simulink model "Elevator"  (R2023b)
settings: Solver=VariableStepAuto  StartTime=0.0  StopTime=inf  RelTol=1e-3
(part 2 of 2)

== matlab function Elevator/MATLAB Function ==
  data: eb input; i1 input; i2 input; i3 input; EBL output; pw input; o1 input; o2 input; o3 input; EL output; VE output; VD output; i_f input; f_t output; c_f output; f output; i_f output; n_f output; i_2 output; i_3 output; i_1 output
function [EBL,EL,VE,VD,f_t,c_f,f,i_f,n_f,i_2,i_3,i_1] = fcn(eb,i1,i2,i3,pw,o1,o2,o3,i_f)



%-----------------------------------------------------------------------------------
if o1 == 1
    f = 1;
elseif o2 == 1 
    f = 2;
elseif o3 == 1  
    f = 3;
else
    f = 0;
end

%------------------------------------------------------------------------------------
if i1==1 && i2==0 && i3==0
    n_f = 1;
elseif i1==0 && i2==1 && i3==0
    n_f = 2;
elseif i1==0 && i2==0 && i3==1
    n_f = 3;
elseif i1==1 && i2==1 && i3==0
    n_f = 4;
elseif i1==1 && i2==0 && i3==1
    n_f = 5;
elseif i1==0 && i2==1 && i3==1
    n_f = 6;
elseif i1==1 && i2==1 && i3==1
    n_f = 7; 
else
    n_f = 0;
end
%-----------------------------------------------------------------------------------
if eb == 1
    EBL = 1;
else 
    EBL = 0;
end
%-----------------------------------------------------------------------------------
if (o1+o2+o3)>=2 || (i1+i2+i3)==0 || (f==n_f)
    EL = 1;
    c_f = 3;
else
    EL = 0;
    c_f = f-i_f;
end
%-----------------------------------------------------------------------------------
VE = pw*0.25;
VD = 86.3;
k=1.02;
f_t = pw*k;
i_1=i1;
i_2=i2;
i_3=i3;
%-----------------------------------------------------------------------------------

%Hamid Reza Heidari - Control Of Mechatronic Systems - AmirKabir University Of Technology - 2023-24-12%

== stateflow chart Elevator/Discrete-Event Chart ==
  settings: enableNonTerminalStates=1
  state Elevator [group]
    state S0
      en:
      Floor = 0 ;
    state EB
      en:
      EBL=1;
      Up=0;
      Down=0;
      Motor_LR_Voltage=0;
      Motor_UD_Voltage=0;
      Switch_LR = 0;
      Switch_UD = 0;
      Floor = 0;
      Door_Open = 0;
      Door_Close = 0;
    state S1
      en:
      Motor_UD_Voltage = VE;
      Switch_UD = 2;
      Up = 1;
      Floor = i_f;
    state S3
      en:
      Floor = f;
      Switch_UD = 1;
    state S2
      en:
      Motor_UD_Voltage = VE;
      Switch_UD = 1;
      Down = 1;
      Floor = i_f;
    state STOP
    state B
      state EB
        en:
        EBL=1;
      state K
      state G
        state EB
        state G0
        state G2
          state B1
            en:Up=1;
          state B2
            en:Up=1;
          state EB1
            en:
            EBL=1;
            Up=0;
            Down=0;
            Motor_LR_Voltage=0;
            Motor_UD_Voltage=0;
            Switch_LR = 0;
            Switch_UD = 0;
            Floor = 0;
            Door_Open = 0;
            Door_Close = 0;
          state B4
            en:
            Floor = 2;
          state B3
            en:
            Floor = 2;
          state Door_Action
            state EB1
            state DA0
              en:
              Switch_UD = 0;
              Motor_UD_Voltage = 0;
            state DA1
              en:
              Door_Open = 1;
              Switch_LR = 1;
              Motor_LR_Voltage = VD;
              Up = 0;
            state DA2
              en:
              Door_Open = 0;
              Motor_LR_Voltage = 0;
            state DA4
              en:
              Up=1;
              Door_Close=0;
              Motor_LR_Voltage = 0;
              Switch_LR = 0;
            state DA3
              en:
              Door_Close=1;
              Switch_LR = 2;
            state DA5
              en:
              Motor_UD_Voltage = VE;
            (default) -> Elevator.B.G.G2.Door_Action.EB1 [order 1] : [EB==1]
            (default) -> Elevator.B.G.G2.Door_Action.DA0 [order 2]
            Elevator.B.G.G2.Door_Action.DA0 -> Elevator.B.G.G2.Door_Action.DA1 : after(285,msec)
            Elevator.B.G.G2.Door_Action.DA1 -> Elevator.B.G.G2.Door_Action.DA2 : after(385,msec)
            Elevator.B.G.G2.Door_Action.DA2 -> Elevator.B.G.G2.Door_Action.DA3 : after(285,msec)
            Elevator.B.G.G2.Door_Action.DA3 -> Elevator.B.G.G2.Door_Action.DA4 : after(385,msec)
            Elevator.B.G.G2.Door_Action.DA4 -> Elevator.B.G.G2.Door_Action.DA5 : after(285,msec)
          state B5
            en:
            Floor = 3;
          (default) -> Elevator.B.G.G2.EB1 [order 2] : [EB==1]
          (default) -> Elevator.B.G.G2.B1 [order 1] : [i3==0]
          (default) -> Elevator.B.G.G2.B2 [order 3]
          Elevator.B.G.G2.B1 -> Elevator.B.G.G2.B4 : after(f_t,msec)
          Elevator.B.G.G2.B2 -> Elevator.B.G.G2.B3 : after(f_t,msec)
          Elevator.B.G.G2.Door_Action.EB1 -> Elevator.B.G.G2.EB1
          Elevator.B.G.G2.B3 -> Elevator.B.G.G2.Door_Action : after(185,msec)
          Elevator.B.G.G2.Door_Action.DA5 -> Elevator.B.G.G2.B5 : after(f_t,msec)
        state G1
          en:Up=1;
        state G5
          en:
          Up=1;
          Floor = 2;
        state G3
          en:
          Floor = 3;
        state G4
        (default) -> Elevator.B.G.EB [order 3] : [EB==1]
        (default) -> Elevator.B.G.G0 [order 4]
        (default) -> Elevator.B.G.G1 [order 1] : [i2==0]
        (default) -> Elevator.B.G.G2 [order 2] : [i2==1]
        Elevator.B.G.G1 -> Elevator.B.G.G5 : after(f_t,msec)
        Elevator.B.G.G5 -> Elevator.B.G.G3 : after(f_t,msec)
        Elevator.B.G.G2.B4 -> Elevator.B.G.G4
        Elevator.B.G.G3 -> Elevator.B.G.G4
        Elevator.B.G.G2.B5 -> Elevator.B.G.G4
      state H
        state EB1
        state G0
        state G2
          state B1
            en:Down=1;
          state B2
            en:Down=1;
          state EB1
            en:
            EBL=1;
            Up=0;
            Down=0;
            Motor_LR_Voltage=0;
            Motor_UD_Voltage=0;
            Switch_LR = 0;
            Switch_UD = 0;
            Floor = 0;
            Door_Open = 0;
            Door_Close = 0;
          state B3
            en:
            Floor = 2;
          state B4
            en:
            Floor = 2;
          state Door_Action
            state EB1
            state DA0
              en:
              Switch_UD = 0;
              Motor_UD_Voltage = 0;
            state DA1
              en:
              Door_Open = 1;
              Switch_LR = 1;
              Motor_LR_Voltage = VD;
              Down = 0;
            state DA2
              en:
              Door_Open = 0;
              Motor_LR_Voltage = 0;
            state DA4
              en:
              Down=1;
              Door_Close=0;
              Motor_LR_Voltage = 0;
              Switch_LR = 0;
            state DA3
              en:
              Door_Close=1;
              Switch_LR = 2;
            state DA5
              en:
              Motor_UD_Voltage = VE;
            (default) -> Elevator.B.H.G2.Door_Action.EB1 [order 1] : [EB==1]
            (default) -> Elevator.B.H.G2.Door_Action.DA0 [order 2]
            Elevator.B.H.G2.Door_Action.DA0 -> Elevator.B.H.G2.Door_Action.DA1 : after(285,msec)
            Elevator.B.H.G2.Door_Action.DA1 -> Elevator.B.H.G2.Door_Action.DA2 : after(385,msec)
            Elevator.B.H.G2.Door_Action.DA2 -> Elevator.B.H.G2.Door_Action.DA3 : after(285,msec)
            Elevator.B.H.G2.Door_Action.DA3 -> Elevator.B.H.G2.Door_Action.DA4 : after(385,msec)
            Elevator.B.H.G2.Door_Action.DA4 -> Elevator.B.H.G2.Door_Action.DA5 : after(285,msec)
          state B5
            en:
            Floor = 1;
          (default) -> Elevator.B.H.G2.EB1 [order 2] : [EB==1]
          (default) -> Elevator.B.H.G2.B1 [order 1] : [i1==0]
          (default) -> Elevator.B.H.G2.B2 [order 3]
          Elevator.B.H.G2.B1 -> Elevator.B.H.G2.B3 : after(f_t,msec)
          Elevator.B.H.G2.B2 -> Elevator.B.H.G2.B4 : after(f_t,msec)
          Elevator.B.H.G2.Door_Action.EB1 -> Elevator.B.H.G2.EB1
          Elevator.B.H.G2.B4 -> Elevator.B.H.G2.Door_Action : after(185,msec)
          Elevator.B.H.G2.Door_Action.DA5 -> Elevator.B.H.G2.B5
        state G1
        state G5
          en:
          Down=1;
          Floor = 2;
        state G3
          en:
          Floor = 1;
        state G4
        (default) -> Elevator.B.H.G1 [order 1] : [i2==0]
        (default) -> Elevator.B.H.EB1 [order 3] : [EB==1]
        (default) -> Elevator.B.H.G0 [order 4]
        (default) -> Elevator.B.H.G2 [order 2] : [i2==1]
        Elevator.B.H.EB1 -> Elevator.B.H.G2.EB1
        Elevator.B.H.G1 -> Elevator.B.H.G5 : after(f_t,msec)
        Elevator.B.H.G5 -> Elevator.B.H.G3 : after(f_t,msec)
        Elevator.B.H.G2.B3 -> Elevator.B.H.G4
        Elevator.B.H.G3 -> Elevator.B.H.G4
        Elevator.B.H.G2.B5 -> Elevator.B.H.G4
      state J
        state J0
        state J5
          en:
          Down=1
        state J1
          en:
          Up=1
        state EB1
          en:
          EBL=1;
          Up=0;
          Down=0;
          Motor_LR_Voltage=0;
          Motor_UD_Voltage=0;
          Switch_LR = 0;
          Switch_UD = 0;
          Floor = 0;
          Door_Open = 0;
          Door_Close = 0;
        state J2
          en:
          Floor = 3;
        state J6
          en:
          Floor = 1;
        state Door_Action1
          state EB1
          state DA0
            en:
            Switch_UD = 0;
            Motor_UD_Voltage = 0;
          state DA1
            en:
            Door_Open = 1;
            Switch_LR = 1;
            Motor_LR_Voltage = VD;
            Up = 0;
          state DA2
            en:
            Door_Open = 0;
            Motor_LR_Voltage = 0;
          state DA4
            en:
            Down=1;
            Door_Close=0;
            Motor_LR_Voltage = 0;
            Switch_LR = 0;
          state DA3
            en:
            Door_Close=1;
            Switch_LR = 2;
          state DA5
            en:
            Motor_UD_Voltage = VE;
          (default) -> Elevator.B.J.Door_Action1.EB1 [order 1] : [EB==1]
          (default) -> Elevator.B.J.Door_Action1.DA0 [order 2]
          Elevator.B.J.Door_Action1.DA0 -> Elevator.B.J.Door_Action1.DA1 : after(285,msec)
          Elevator.B.J.Door_Action1.DA1 -> Elevator.B.J.Door_Action1.DA2 : after(385,msec)
          Elevator.B.J.Door_Action1.DA2 -> Elevator.B.J.Door_Action1.DA3 : after(285,msec)
          Elevator.B.J.Door_Action1.DA3 -> Elevator.B.J.Door_Action1.DA4 : after(385,msec)
          Elevator.B.J.Door_Action1.DA4 -> Elevator.B.J.Door_Action1.DA5 : after(285,msec)
        state Door_Action2
          state EB1
          state DA0
            en:
            Switch_UD = 0;
            Motor_UD_Voltage = 0;
          state DA1
            en:
            Door_Open = 1;
            Switch_LR = 1;
            Motor_LR_Voltage = VD;
            Down = 0;
          state DA2
            en:
            Door_Open = 0;
            Motor_LR_Voltage = 0;
          state DA4
            en:
            Up=1;
            Door_Close=0;
            Motor_LR_Voltage = 0;
            Switch_LR = 0;
          state DA3
            en:
            Door_Close=1;
            Switch_LR = 2;
          state DA5
            en:
            Motor_UD_Voltage = VE;
          (default) -> Elevator.B.J.Door_Action2.EB1 [order 1] : [EB==1]
          (default) -> Elevator.B.J.Door_Action2.DA0 [order 2]
          Elevator.B.J.Door_Action2.DA0 -> Elevator.B.J.Door_Action2.DA1 : after(285,msec)
          Elevator.B.J.Door_Action2.DA1 -> Elevator.B.J.Door_Action2.DA2 : after(385,msec)
          Elevator.B.J.Door_Action2.DA2 -> Elevator.B.J.Door_Action2.DA3 : after(285,msec)
          Elevator.B.J.Door_Action2.DA3 -> Elevator.B.J.Door_Action2.DA4 : after(385,msec)
          Elevator.B.J.Door_Action2.DA4 -> Elevator.B.J.Door_Action2.DA5 : after(285,msec)
        state J3
          en:
          Floor = 2;
        state J7
          en:
          Floor = 2;
        state J4
          en:
          Floor = 1;
        state J8
          en:
          Floor = 3;
        state J9
        (default) -> J1 [order 1] : [Switch_UD == 2]
        (default) -> J5 [order 2] : [Switch_UD == 1]
        (default) -> J0 [order 4]
        (default) -> Elevator.B.J.EB1 [order 3] : [EB==1]
        J5 -> J6 : after(f_t,msec)
        J1 -> J2 : after(f_t,msec)
        Elevator.B.J.Door_Action2.EB1 -> Elevator.B.J.EB1
        J2 -> Door_Action1
        Elevator.B.J.Door_Action1.EB1 -> Elevator.B.J.EB1
        J6 -> Door_Action2
        Elevator.B.J.Door_Action1.DA5 -> J3
        Elevator.B.J.Door_Action2.DA5 -> J7
        J3 -> J4 : after(f_t,msec)
        J7 -> J8 : after(f_t,msec)
        J4 -> J9
        J8 -> J9
      (default) -> Elevator.B.EB [order 6] : [EB==1]
      (default) -> K [order 7]
      Elevator.B.EB -> Elevator.B.J.EB1
      (default) -> G [order 2] : [f==1]
      (default) -> J [order 1] : [f==2 && (n_f ==5 || n_f == 7) ]
      (default) -> H [order 4] : [f==3]
      (default) -> Elevator.B.G.G5 [order 3] : [f==2 && (n_f == 3 || n_f == 6) ]
      (default) -> Elevator.B.H.G5 [order 5] : [f==2 && (n_f == 2 || n_f == 4) ]
    state A
      state EB1
        en:
        EBL=1;
        Up=0;
        Down=0;
        Motor_LR_Voltage=0;
        Motor_UD_Voltage=0;
        Switch_LR = 0;
        Switch_UD = 0;
        Floor = 0;
        Door_Open = 0;
        Door_Close = 0;
      state S4
        en:
        if c_f>0
        Floor = c_f;
        else
        Floor = -1*(c_f)
        end
      state S5
        en:
        Floor = f ;
      state Door_Action
        state EB1
        state DA0
          en:
          Motor_UD_Voltage = 0;
        state DA1
          en:
          Door_Open = 1;
          Switch_LR = 1;
          Motor_LR_Voltage = VD;
          Up = 0;
          Down=0;
        state DA2
          en:
          Door_Open = 0;
          Motor_LR_Voltage = 0;
        state DA4
          en:
          Door_Close=0;
          Motor_LR_Voltage = 0;
          Switch_LR = 0;
        state DA3
          en:
          Door_Close=1;
          Switch_LR = 2;
        state DA5
          en:
          Motor_UD_Voltage = VE;
        (default) -> Elevator.A.Door_Action.EB1 [order 1] : [EB==1]
        (default) -> Elevator.A.Door_Action.DA0 [order 2]
        Elevator.A.Door_Action.DA0 -> Elevator.A.Door_Action.DA1 : after(285,msec)
        Elevator.A.Door_Action.DA1 -> Elevator.A.Door_Action.DA2 : after(385,msec)
        Elevator.A.Door_Action.DA2 -> Elevator.A.Door_Action.DA3 : after(285,msec)
        Elevator.A.Door_Action.DA3 -> Elevator.A.Door_Action.DA4 : after(385,msec)
        Elevator.A.Door_Action.DA4 -> Elevator.A.Door_Action.DA5 : after(285,msec)
      (default) -> Elevator.A.EB1 [order 2] : [EB==1]
      (default) -> S5 [order 1] : [c_f==1 || c_f==-1]
      (default) -> S4 [order 4]
      S4 -> S5 : after(f_t,msec)
      S5 -> Elevator.A.Door_Action : after(185,msec)
      Elevator.A.Door_Action.EB1 -> Elevator.A.EB1
      (default) -> Elevator.A.Door_Action [order 3] : [c_f==0]
    state Door_Action
      state DA0
        en:
        Switch_UD = 0;
        Motor_UD_Voltage = 0;
      state DA1
        en:
        Door_Open = 1;
        Switch_LR = 1;
        Motor_LR_Voltage = VD;
        Down = 0;
        Up=0;
      state DA2
        en:
        Door_Open = 0;
        Motor_LR_Voltage = 0;
      state DA4
        en:
        Door_Close=0;
        Motor_LR_Voltage = 0;
        Switch_LR = 0;
      state DA3
        en:
        Door_Close=1;
        Switch_LR = 2;
      state EB1
        en:
        EBL=1;
        Up=0;
        Down=0;
        Motor_LR_Voltage=0;
        Motor_UD_Voltage=0;
        Switch_LR = 0;
        Switch_UD = 0;
        Floor = 0;
        Door_Open = 0;
        Door_Close = 0;
      (default) -> Elevator.Door_Action.DA0 [order 2]
      Elevator.Door_Action.DA0 -> Elevator.Door_Action.DA1 : after(285,msec)
      Elevator.Door_Action.DA1 -> Elevator.Door_Action.DA2 : after(385,msec)
      Elevator.Door_Action.DA2 -> Elevator.Door_Action.DA3 : after(285,msec)
      (default) -> Elevator.Door_Action.EB1 [order 1] : [EB==1]
      Elevator.Door_Action.DA3 -> Elevator.Door_Action.DA4 : after(385,msec)
    (default) -> S3 [order 4] : [c_f==0]
    (default) -> Elevator.EB [order 5] : [EB==1]
    (default) -> S1 [order 1] : [c_f>0 && c_f<3]
    (default) -> S2 [order 2] : [c_f<0]
    (default) -> S0 [order 3] : [c_f ==3]
    (default) -> STOP [order 6]
    S2 -> A : after(f_t,msec)
    S3 -> A : after(175,msec)
    S1 -> A : after(f_t,msec)
    Elevator.B.G.G4 -> Elevator.Door_Action : after(185,msec)
    Elevator.A.Door_Action.DA5 -> B : after(185,msec)
    Elevator.B.H.G4 -> Elevator.Door_Action : after(185,msec)
    J9 -> Elevator.Door_Action : after(185,msec)
  data: EB input; c_f input; f_t input; Floor output double; Switch_LR output; Up output; Door_Open output; Down output; Motor_LR_Voltage output; Motor_UD_Voltage output; Switch_UD output; VE input; VD input; f input; i_f input; n_f input; Door_Close output; i2 input; i3 input; i1 input; EBL output
